simulink model "new_my_brake_system"  (R2024a)
settings: Solver=ode45  StartTime=0  StopTime=2000  FixedStep=.001  RelTol=1e-3  EnableMultiTasking=on
model workspace (MAT data in the model file):
  J = 0.226199211484
  Kt = 174.53
  Ts_verif = Simulink.Parameter
  Ts_verif.Value = 0.001
  Ts_verif.Complexity = 'real'
  Ts_verif.Dimensions = [1 1]
  Ts_verif.DataType = 'auto'
  angle_init = 15
  angle_open = 85
  c = 8.89069171842
  fall_end_angle = Simulink.Parameter
  fall_end_angle.Value = 0.1
  fall_end_angle.Complexity = 'real'
  fall_end_angle.Dimensions = [1 1]
  fall_end_angle.DataType = 'auto'
  fall_start_angle = Simulink.Parameter
  fall_start_angle.Value = 0.9
  fall_start_angle.Complexity = 'real'
  fall_start_angle.Dimensions = [1 1]
  fall_start_angle.DataType = 'auto'
  input_delay = 0.00986306560803
  k = 19.1559540807
  rise_end_angle = Simulink.Parameter
  rise_end_angle.Value = 0.9
  rise_end_angle.Complexity = 'real'
  rise_end_angle.Dimensions = [1 1]
  rise_end_angle.DataType = 'auto'
  rise_start_angle = Simulink.Parameter
  rise_start_angle.Value = 0.1
  rise_start_angle.Complexity = 'real'
  rise_start_angle.Dimensions = [1 1]
  rise_start_angle.DataType = 'auto'
  vv_fall_time_max = Simulink.Parameter
  vv_fall_time_max.Value = 0.3
  vv_fall_time_max.Complexity = 'real'
  vv_fall_time_max.Dimensions = [1 1]
  vv_fall_time_max.DataType = 'auto'
  vv_fall_time_min = Simulink.Parameter
  vv_fall_time_min.Value = 0.001
  vv_fall_time_min.Complexity = 'real'
  vv_fall_time_min.Dimensions = [1 1]
  vv_fall_time_min.DataType = 'auto'
  vv_rise_time_max = Simulink.Parameter
  vv_rise_time_max.Value = 0.1
  vv_rise_time_max.Complexity = 'real'
  vv_rise_time_max.Dimensions = [1 1]
  vv_rise_time_max.DataType = 'auto'
  vv_rise_time_min = Simulink.Parameter
  vv_rise_time_min.Value = 0.001
  vv_rise_time_min.Complexity = 'real'
  vv_rise_time_min.Dimensions = [1 1]
  vv_rise_time_min.DataType = 'auto'
(part 1 of 2)
settings Model: Creator=The MathWorks, Inc.  LastModifiedBy=Mhamed
settings SolverCC: AlgebraicLoopSolver=TrustRegion  AutoInsertRateTranBlk=on
settings DataIOCC: SaveFormat=Array  SaveOutput=off  SaveTime=off  ReturnWorkspaceOutputs=off  SignalLoggingName=DataLog
settings OptimizationCC: BooleanDataType=off  DefaultParameterBehavior=Inlined  InlineInvariantSignals=on  ExpressionDepthLimit=2147483647  InitFltsAndDblsToZero=on  NoFixptDivByZeroProtection=on  EfficientFloat2IntCast=on  LifeSpan=1  BufferReusableBoundary=off  EfficientTunableParamExpr=on
settings DebuggingCC: SaveWithParameterizedLinksMsg=none  SignalResolutionControl=TryResolveAll  MultiTaskDSMMsg=warning  IntegerOverflowMsg=none  ParameterOverflowMsg=warning  ParameterPrecisionLossMsg=none  FcnCallInpInsideContextMsg=warning  UnconnectedInputMsg=warning  UnconnectedOutputMsg=warning  UnconnectedLineMsg=warning  BusObjectLabelMismatch=none  StateNameClashWarn=warning  SFUnexpectedBacktrackingDiag=warning  SFNoUnconditionalDefaultTransitionDiag=warning  SFExecutionAtInitializationDiag=none  ArithmeticOperatorsInVariantConditions=warning
settings HardwareCC: ProdBitPerPointer=32  ProdBitPerSizeT=32  ProdBitPerPtrDiffT=32  ProdLargestAtomicFloat=None  ProdIntDivRoundTo=Undefined  ProdEndianess=Unspecified  ProdWordSize=32  ProdHWDeviceType=32-bit Generic
settings ModelReferenceCC: EnableRefExpFcnMdlSchedulingChecks=on  PropagateSignalLabelsOutOfModel=off
settings SFSimCC: SimUseLocalCustomCode=off  SimParseCustomCode=off  MATLABDynamicMemAlloc=off  CustomCodeUndefinedFunction=UseInterfaceOnly
settings RTWCC: Description=Real-Time Workshop Embedded Coder (no auto configuration)  SystemTargetFile=ert.tlc  TemplateMakefile=ert_default_tmf  GenerateReport=on  RTWUseLocalCustomCode=off  IncludeHyperlinkInReport=on  LaunchReport=on  GPUComputeCapability=3.5  DLArmComputeVersion=19.05
settings CodeAppCC: IgnoreCustomStorageClasses=off  SimulinkDataObjDesc=on  CustomSymbolStrType=$N$R$M  StateflowObjectComments=on  InternalIdentifier=Classic  ReqsInCode=on
settings ERTTargetCC: TargetFcnLib=ansi_tfl_tmw.mat  UtilityFuncGeneration=Shared location  MultiwordLength=2048  GenerateSampleERTMain=on  IncludeMdlTerminateFcn=off  SuppressErrorStatus=on  SupportAbsoluteTime=off  SupportNonFinite=off  SupportComplex=off  InlinedParameterPlacement=NonHierarchical  ERTSrcFileBannerTemplate=eng_ctrl_code_template.cgt  ERTCustomFileTemplate=example_file_process.tlc  ConvertIfToSwitch=off  SuppressUnreachableDefaultCases=off
settings ConfigComp: CovMetricSettings=dw  CovSaveCumulativeToWorkspaceVar=on  CovSaveSingleToWorkspaceVar=on  CovExternalEMLEnable=off
settings SimscapeCC: SimscapeNormalizeSystem=off

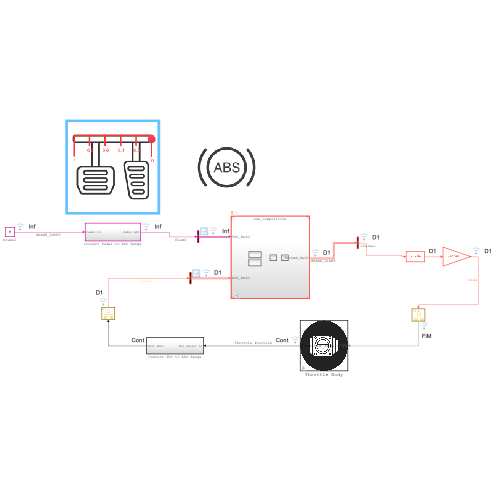
[thumbnail: Simulink's stored preview of the top-level diagram]
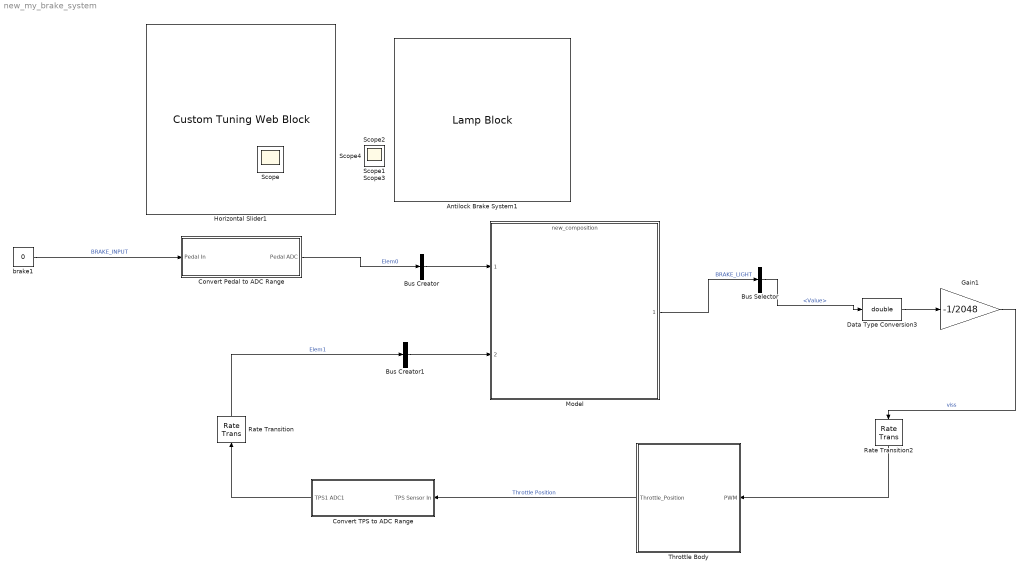
== system new_my_brake_system ==
  Antilock Brake System1 : LampBlock  LabelPosition=Hide  Icon=AntilockBrakeSystem
  Bus Creator : BusCreator  Inputs=1
  Bus Creator1 : BusCreator  Inputs=1
  Bus Selector : BusSelector  OutputSignals=Value
  Convert Pedal to ADC Range : Subsystem
  Convert TPS to ADC Range : Subsystem
  Data Type Conversion3 : DataTypeConversion  OutDataTypeStr=double  SaturateOnIntegerOverflow=off  RndMeth=Floor
  Gain1 : Gain  Gain=-1/2048
  Horizontal Slider1 : CustomTuningWebBlock  LabelPosition=Hide  ShowInitialText=on  Configuration="{\"components\":[{\"name\":\"LinearScaleComponent\",\"settings\":{\"bounds\":{\"max\":1,\"min\":0,\"tickInterval\":\"auto\"},\"internalTickHeightScaleFactor\":0.5,\"labelColor\":[255,0,0],\"labelFont\":{\"font\":\"Arial\",\"fontSize\":12},\"labelOffset\":0.05,\"labelTransparency\":1,\"needleImage\":{\"size\":[200,200],\"src\":\"data:image\\/png;base64,iVBORw0KGgoAAAANSUhEUgAAAMgAAADICAYAAACtWK6eAAAABGdBTUEAALGPC\\/xhBQAAACBjSFJNAAB6JgAAgIQAAPoAAACA6AAAdTAAAOpgAAA6mAAAF3CculE8AAAABmJLR0QA\\/wD\\/AP+gvaeTAAAACXBIWXMAAAsSAAALEgHS3X78AAAAB3RJTUUH5gsWCQ4Mlo8xRwAAFzJJREFUeNrtnXuwJVdVh7++987jZh7JvGfyGiYhZAixJo+ZjFGBCFgmGlEExVSlpCwFtAilJRWhEPlHQQGpEpEylFhapiyLN1GpUEIMiCWaYCAJJJPEvIZk8s5kZu7cmblz5yz\\/2N2nd3fvvXv3OWfm3u6zvplzbvfuvXf36V6\\/s9ba3acbFEVRFE ...(+8098 chars)\",\"srcOrientation\":\"Right\"},\"needleOffset\":[-0.2610466535701308,-0.059006590280473586],\"needleSize\":{\"height\":0.1829787234042553,\"width\":0.17127659574468085},\"position\":[0.09142287234042554,0.022606382978723406,0.9674866858949053,0.37473406690232297],\"referencePoint\":\"auto\",\"scaleColors\":[],\"scaleColorsSize\":0.2,\"scaleDirection\":\"RL\",\"showLabels\":1,\"showMinorTicks\":0,\"showSpanLine\":1,\"showTicks\":1,\"tickColor\":[255,0,0],\"tickTransparency\":1,\"valueBarColor\":[255,0,0],\"valueBarOffset\":-0.27,\"valueBarSize\":0.1,\"valueBarTransparency\":1}},{\"name\":\"BackgroundImageComponent\",\"settings\":{\"image\":{\"size\":[740,740],\"src\":\"data:image\\/jpeg;base64,\\/9j\\/4AAQSkZJRgABAQAAAAAAAAD\\/2wBDAAQDAwQDAwQEAwQFBAQFBgoHBgYGBg0JCggKDw0QEA8NDw4RExgUERIXEg4PFRwVFxkZGxsbEBQdHx0aHxgaGxr\\/wgALCALkAuQBASIA\\/8QAHAABAAEFAQEAAAAAAAAAAAAAAAgBBAUGBwID\\/9oACAEBAAAAAe\\/gAAAAAAAAAAAAAAAAAAAAAAAAAAAAAAAAAAAAAAAAAAAAAAAAAAAAAAAAAAAAAAAAAAAAAAAAAAAAAAAAAAAAAAAAAAAAAAAAAAAAAAAAAAAAAAAAAAAAAAAAAAAAAAAAAAAAAAAAAAAAAAAAAAAAAAAAAAAAAAAAAAAAAAAAAAAAAAAAAAAAAAAAAA1bQPn9vl ...(+45306 chars)\",\"srcOrientation\":\"Right\"},\"position\":[0,0,1,1],\"scaleMode\":\"0\"}},{\"name\":\"ForegroundImageComponent\",\"settings\":{\"image\":{\"size\":[0,0],\"src\":\"default\",\"srcOrientation\":[]},\"isForeground\":1,\"position\":[0,0,1,1],\"scaleMode\":\"0\"}}],\"settings\":{\"BindingType\":\"param\",\"aspectRatio\":3.7777777777777777,\"backgroundColor\":[0,0,0,\"1\"],\"backgroundOffset\":0,\"backgroundOpacity\":1,\"fixedAspectRatio\":\"on\",\"foregroundColor\":[252,252,196],\"orientation\":\"horizontal\",\"showBackgroundColor\":false,\"value\":0,\"version\":\"R2023a\"},\"type\":\"LinearGauge\"}"
  Model : ModelReference  ModelNameDialog=new_composition.slx  SimulationMode=Normal  ScheduleRates=on  ScheduleRatesWith=Schedule Editor  ModelReferenceVersion=1.7
  Rate Transition : RateTransition  Deterministic=off  OutPortSampleTime=.005
  Rate Transition2 : RateTransition  Deterministic=off
  Throttle Body : Subsystem  mask{units=normalized, input_delay=input_delay, J=J, c=c, k=k, close_angle=angle_init, open_angle=angle_open}
      mask prompts: input_delay "Input Delay:"; J "Inertia:"; c "Damping:"; k "Stiffness:"; close_angle "Resting Angle:"; open_angle "Open Angle:"
      mask TypeOptions units: rads | degrees | normalized
      mask Display: image('throttle-plate-icon-vector.jpg');
  brake1 : Constant  Value=0  OutMin=0  OutMax=1  OutDataTypeStr=uint16
  Scope{,1..4} (5 alike) : Scope
  wires:
  Rate Transition2/1 -> Throttle Body/1(PWM)
  Data Type Conversion3/1 -> Gain1/1
  Throttle Body/1(Throttle_Position) -> Convert TPS to ADC Range/1(TPS Sensor In)  "Throttle Position"
  Convert TPS to ADC Range/1(TPS1 ADC1) -> Rate Transition/1
  brake1/1 -> Convert Pedal to ADC Range/1(Pedal In)  "BRAKE_INPUT"
  Gain1/1 -> Rate Transition2/1  "viss"
  Bus Selector/1 -> Data Type Conversion3/1  "<Value>"
  Model/1 -> Bus Selector/1  "BRAKE_LIGHT"
  Bus Creator1/1 -> Model/2
  Rate Transition/1 -> Bus Creator1/1  "Elem1"
  Bus Creator/1 -> Model/1
  Convert Pedal to ADC Range/1(Pedal ADC) -> Bus Creator/1  "Elem0"
